simulink model "humdifer"  (R2014b)
settings: Solver=ode45  StartTime=0.0  StopTime=10.0  RelTol=1e-3
settings Model: Creator=dell  LastModifiedBy=dell

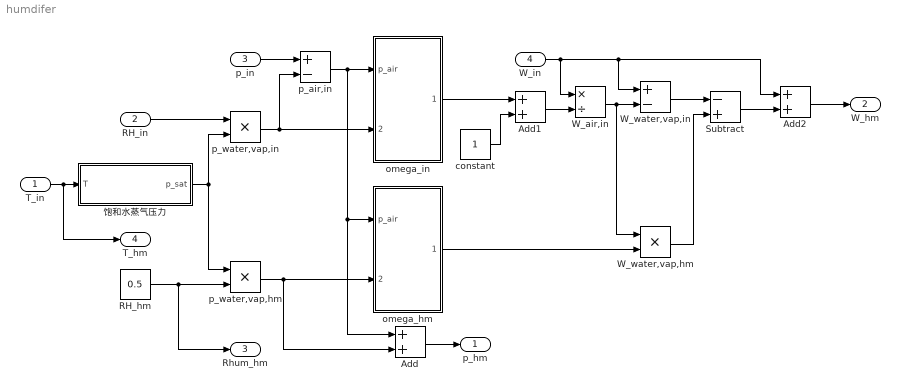
== system humdifer ==
  T_in : Inport
  RH_in : Inport  Port=2
  p_in : Inport  Port=3
  W_in : Inport  Port=4
  Add : Sum
  Add1 : Sum
  Add2 : Sum
  RH_hm : Constant  Value=0.5
  Subtract : Sum  Inputs=-+
  W_air,in : Product  Inputs=*/
  W_water,vap,hm : Product
  W_water,vap,in : Sum  Inputs=+-
  "constant " : Constant
  omega_hm : Subsystem
  omega_in : Subsystem
  p_air,in : Sum  Inputs=+-
  p_water,vap,hm : Product
  p_water,vap,in : Product
  饱和水蒸气压力 : Subsystem
  p_hm : Outport
  W_hm : Outport  Port=2
  Rhum_hm : Outport  Port=3
  T_hm : Outport  Port=4
  wires:
  T_in/1 -> T_hm/1, 饱和水蒸气压力/1(T)
  饱和水蒸气压力/1(p_sat) -> p_water,vap,hm/1, p_water,vap,in/2
  RH_hm/1 -> p_water,vap,hm/2, Rhum_hm/1
  RH_in/1 -> p_water,vap,in/1
  p_water,vap,in/1 -> omega_in/2(p_water), p_air,in/2
  p_in/1 -> p_air,in/1
  p_air,in/1 -> omega_in/1(p_air), omega_hm/1(p_air), Add/1
  p_water,vap,hm/1 -> omega_hm/2(p_water), Add/2
  Add/1 -> p_hm/1
  omega_in/1(omega) -> Add1/1
  "constant "/1 -> Add1/2
  Add1/1 -> W_air,in/2
  W_in/1 -> W_air,in/1, W_water,vap,in/1, Add2/1
  W_air,in/1 -> W_water,vap,in/2, W_water,vap,hm/1
  omega_hm/1(omega) -> W_water,vap,hm/2
  W_water,vap,in/1 -> Subtract/1
  W_water,vap,hm/1 -> Subtract/2
  Subtract/1 -> Add2/2
  Add2/1 -> W_hm/1

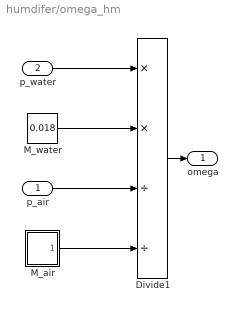
== system humdifer/omega_hm ==
  p_air : Inport
  p_water : Inport  Port=2
  Divide1 : Product  Inputs=**//
  M_air : Subsystem
  M_water : Constant  Value=0.018
  omega : Outport
  wires:
  M_water/1 -> Divide1/2
  p_air/1 -> Divide1/3
  M_air/1(M_air) -> Divide1/4
  p_water/1 -> Divide1/1
  Divide1/1 -> omega/1

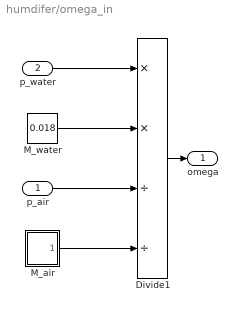
== system humdifer/omega_in ==
  p_air : Inport
  p_water : Inport  Port=2
  Divide1 : Product  Inputs=**//
  M_air : Subsystem
  M_water : Constant  Value=0.018
  omega : Outport
  wires:
  M_water/1 -> Divide1/2
  p_air/1 -> Divide1/3
  M_air/1(M_air) -> Divide1/4
  p_water/1 -> Divide1/1
  Divide1/1 -> omega/1

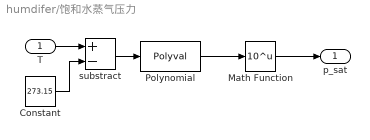
== system humdifer/饱和水蒸气压力 ==
  T : Inport
  Constant : Constant  Value=273.15
  Math Function : Math  Operator=10^u  SaturateOnIntegerOverflow=on
  Polynomial : Polyval  Coefs=[1.4454e-7,-9.1837e-5,0.2953,-2.1794]
  substract : Sum  Inputs=+-
  p_sat : Outport
  wires:
  Polynomial/1 -> Math Function/1
  T/1 -> substract/1
  Math Function/1 -> p_sat/1
  substract/1 -> Polynomial/1
  Constant/1 -> substract/2

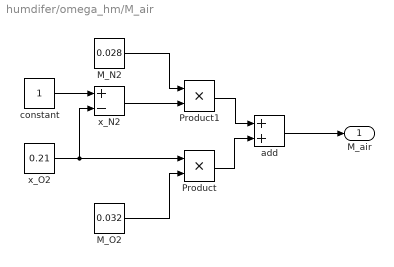
== system humdifer/omega_hm/M_air ==
  M_N2 : Constant  Value=0.028
  M_O2 : Constant  Value=0.032
  Product : Product
  Product1 : Product
  add : Sum
  constant : Constant
  x_N2 : Sum  Inputs=+-
  x_O2 : Constant  Value=0.21
  M_air : Outport
  wires:
  constant/1 -> x_N2/1
  x_O2/1 -> Product/1, x_N2/2
  M_O2/1 -> Product/2
  M_N2/1 -> Product1/1
  x_N2/1 -> Product1/2
  Product/1 -> add/2
  Product1/1 -> add/1
  add/1 -> M_air/1

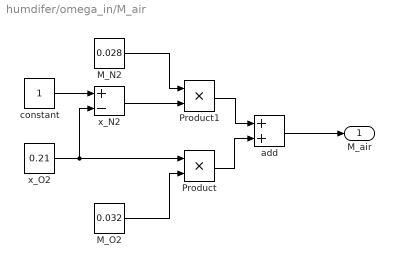
== system humdifer/omega_in/M_air ==
  M_N2 : Constant  Value=0.028
  M_O2 : Constant  Value=0.032
  Product : Product
  Product1 : Product
  add : Sum
  constant : Constant
  x_N2 : Sum  Inputs=+-
  x_O2 : Constant  Value=0.21
  M_air : Outport
  wires:
  constant/1 -> x_N2/1
  x_O2/1 -> Product/1, x_N2/2
  M_O2/1 -> Product/2
  M_N2/1 -> Product1/1
  x_N2/1 -> Product1/2
  Product/1 -> add/2
  Product1/1 -> add/1
  add/1 -> M_air/1
